simulink model "DC_motor_LQR_precomp"  (R2015b)
settings: Solver=VariableStepAuto  StartTime=0.0  StopTime=10  MaxStep=1e-2  RelTol=1e-3
settings Model: Creator=mgreiff  LastModifiedBy=mgreiff
settings DebuggingCC: AlgebraicLoopMsg=none

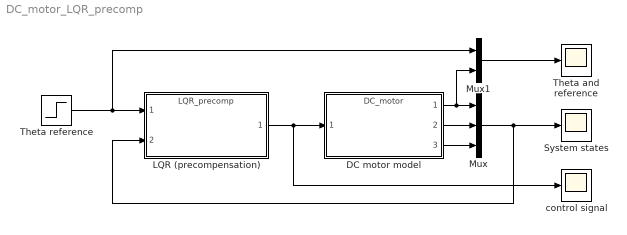
== system DC_motor_LQR_precomp ==
  DC motor model : ModelReference  ModelNameDialog=DC_motor.slx  SimulationMode=Normal  ModelReferenceVersion=1.4  CopyOfModelName=DC_motor.slx
  LQR (precompensation) : ModelReference  ModelNameDialog=LQR_precomp.slx  SimulationMode=Normal  ModelReferenceVersion=1.4  CopyOfModelName=LQR_precomp.slx
  Mux : Mux  Inputs=3
  Mux1 : Mux  Inputs=2
  System states : Scope
  Theta and reference : Scope
  Theta reference : Step  Time=0  SampleTime=0
  control signal : Scope
  wires:
  DC motor model/1 -> Mux1/2, Mux/1
  DC motor model/2 -> Mux/2
  DC motor model/3 -> Mux/3
  Mux/1 -> LQR (precompensation)/2, System states/1
  Theta reference/1 -> LQR (precompensation)/1, Mux1/1
  Mux1/1 -> Theta and reference/1
  LQR (precompensation)/1 -> DC motor model/1, control signal/1
